simulink model "mainController19a"  (R2019a)
settings: Solver=ode3  StartTime=0  StopTime=inf  FixedStep=0.1  RelTol=1e-3
model workspace (MAT data in the model file):
  SL_ROS_VariableLengthArrays_MaxSizes : struct (value not decoded)
values from neighbouring files (symbols this model uses):
  numJoints = MotominiParams.numJoints    [showCompleteDemo.m]
  numPoints = size(Q,2)-2    [showCompleteDemo.m]
undefined symbols (not defined in the file or in its folder): homeToIdleSpline, idleToHomeSpline, Position, Position_SL_Info, Positions, Positions_SL_Info, TimeFromStart, Velocities, Velocities_SL_Info
libraries: robotlib x18, visiontextngfix x3, simulink x2, visionsinks x1
(part 2 of 2)

== matlab function mainController19a/Motion Planner/Planner Response/Joint Trajectory to Spline Matrices/pointsToSplineData ==
  data: pointsMsg input; Q output double size=[numJoints, numPoints+2]; dQ output double size=[numJoints, numPoints+2]; t output double size=[1, numPoints+2]; numJoints parameter; numPoints parameter; isValid output boolean size=[1]
function [Q,dQ,t, isValid] = pointsMsgToSplineData(pointsMsg,numJoints,numPoints)
% Author: Carlos Santacruz-Rosero, Ph.D.
% Copyright 2016 The MathWorks, Inc.

points = pointsMsg(1:numPoints+2);

Q = zeros(numJoints, numPoints+2);
dQ = zeros(numJoints, numPoints+2);
t = zeros(1,numPoints+2);
isValid = true;

numRxJoints = points(1).Positions_SL_Info.CurrentLength;

if numRxJoints ~= numJoints
    isValid = false;
end

for ii = 1:(numPoints+2)
    Q(:,ii) = points(ii).Positions(1:numJoints);
    dQ(:,ii) = points(ii).Velocities(1:numJoints);
    dur = points(ii).TimeFromStart;
    t(ii) =  double(dur.Sec)+double(dur.Nsec)*10^-9;
end

== stateflow chart mainController19a/State Controller/State Controller ==
  state Home
    state Home
      entry:
      requestTrajController = false;
      requestGripController = false;
      plannerRequest= false;
      droppingPos = [0.05;0.2;0.1];
      gripperOpenPos = [0.050; 0.050];
      gripperClosedPos =[0; 0];
    state GoingToHome
      entry:
      % move arm
      requestTrajController = true;
      Qspline = idleToHomeSpline.Q;
      dQspline = idleToHomeSpline.dQ;
      tSpline = idleToHomeSpline.t;
      goalSpline = idleToHomeSpline.Q(:,end);
      % close gripper
      requestGripController = true;
      gripCommand = [0; 0];
      during: % Going To Target
      requestTrajController = false;
      requestGripController = false;
    (default) -> Home.Home
    (junction 80) -> Home.Home
    GoingToHome -> (junction 80) : [goalReached && qActIsValid]
  state Idle
    state GoingToIdle
      entry:
      % move arm
      requestTrajController = true;
      Qspline = homeToIdleSpline.Q;
      dQspline = homeToIdleSpline.dQ;
      tSpline = homeToIdleSpline.t;
      goalSpline = homeToIdleSpline.Q(:,end);
      % open gripper
      requestGripController = true;
      gripCommand = gripperOpenPos;
      during: % Going To Target
      requestTrajController = false;
      requestGripController = false;
    state Idle
      entry:
      objectDetected = uint32(0);
      objectDetectedPos = zeros(3,1);
      % open gripper
      requestGripController = true;
      gripCommand = gripperOpenPos;
      during:
      [objectDetected, objectDetectedPos,droppingPos] = isObjectInScene(detectorPredictedLabels, detectorXYZPoints)
      requestGripController = false;
    GoingToIdle -> Idle.Idle : [goalReached && qActIsValid]
  state Grabbing
    state RequestGrabbingPlan
      entry:
      plannerRequest= true;
      requestTrajController=false;
      plannerObjectID = objectDetected;
      plannerPos = [objectDetectedPos(1);
      objectDetectedPos(2);
      0.018];
      during:
      plannerRequest= false;
      exit:
    state GoingToApproachPoint
      entry:
      requestTrajController = true;
      Qspline = plannerQ;
      dQspline = plannerDQ;
      tSpline = plannerT;
      goalSpline = plannerQ(:,end);
      during: % Going To Target
      requestTrajController = false;
    state RequestApproachingPlan
      entry:
      plannerRequest= true;
      plannerObjectID = objectDetected;
      plannerPos = [objectDetectedPos(1);
      objectDetectedPos(2);
      objectDetectedPos(3)+0.03];
      during:
      plannerRequest= false;
    state DroppingObject
      entry:
      requestGripController = true;
      gripCommand = gripperOpenPos;
      during: % Going To Target
      requestGripController = false;
    state GoingToObject
      entry:
      requestTrajController = true;
      Qspline = plannerQ;
      dQspline = plannerDQ;
      tSpline = plannerT;
      goalSpline = plannerQ(:,end);
      during: % Going To Target
      requestTrajController = false;
    state RequestLeavingPlan
      entry:
      plannerRequest= true;
      plannerObjectID = objectDetected;
      plannerPos = [objectDetectedPos(1);
      objectDetectedPos(2);
      objectDetectedPos(3)+0.1];
      during:
      plannerRequest= false;
      exit:
    state GrabbingObject
      entry:
      gripCommand = gripperClosedPos;
      requestGripController = true;
      during: % Going To Target
      requestGripController = false;
    state GoingToLeavingPoint
      entry:
      requestTrajController = true;
      Qspline = plannerQ;
      dQspline = plannerDQ;
      tSpline = plannerT;
      goalSpline = plannerQ(:,end);
      during: % Going To Leaving Point
      requestTrajController = false;
    state GoingToDroppingPoint
      entry:
      requestTrajController = true;
      Qspline = plannerQ;
      dQspline = plannerDQ;
      tSpline = plannerT;
      goalSpline = plannerQ(:,end);
      during: % Going To Target
      requestTrajController = false;
    state RequestDroppingPlan
      entry:
      plannerRequest= true;
      plannerObjectID = objectDetected;
      plannerPos = droppingPos;
      during:
      plannerRequest= false;
    RequestGrabbingPlan -> GoingToObject : [plannerHasReplied && ...
        | plannerIsValid]
    RequestApproachingPlan -> GoingToApproachPoint : [plannerHasReplied && ...
        | plannerIsValid]
    GoingToApproachPoint -> RequestGrabbingPlan : [goalReached && qActIsValid]
    GoingToDroppingPoint -> DroppingObject : [goalReached && qActIsValid]
    GoingToObject -> GrabbingObject : [goalReached && qActIsValid]
    GrabbingObject -> RequestLeavingPlan : [~isGripperOpen]
    RequestLeavingPlan -> GoingToLeavingPoint : [plannerHasReplied && ...
        | plannerIsValid]
    RequestDroppingPlan -> GoingToDroppingPoint : [plannerHasReplied && ...
        | plannerIsValid]
    GoingToLeavingPoint -> RequestDroppingPlan : [goalReached && qActIsValid]
  Home.Home -> Idle.Idle : [armCommand==1]
  (default) -> Home
  DroppingObject -> GoingToIdle : [isGripperOpen]
  Idle.Idle -> GoingToHome [order 1] : [armCommand == 0]
  Idle.Idle -> RequestApproachingPlan [order 2] : [(objectDetected ~=0) && qActIsValid]
  data: objDetected function_output uint32; objPos function_output; labels function_input uint32; points function_input double; dropPos function_output; armCommand input uint32; detectorPredictedLabels input uint32 size=[10 1]; detectorXYZPoints input double size=[10 3]; plannerHasReplied input boolean size=[1]; plannerQ input double; plannerDQ input double; plannerT input double; plannerIsValid input boolean; qActIsValid input boolean; plannerRequest output boolean size=[1]; plannerPos output double size=[3]; plannerObjectID output uint32 size=[1]; requestTrajController output boolean size=[1]; Qspline output double; dQspline output double; tSpline output; goalReached input boolean; homeToIdleSpline parameter; idleToHomeSpline parameter; requestGripController output boolean; gripCommand output double size=[2 1]; goalSpline output double size=[numJoints,1] =zeros(numJoints,1); gripperOpenPos local =[0.025;0.025]; gripperClosedPos local =[0;0]; droppingPos local; objectDetected local uint32 size=[1]; objectDetectedPos local double size=[3]; data1 local; isGripperOpen input
  function [objDetected,objPos,dropPos] = isObjectInScene(labels, points):
    | function [objDetected,objPos,dropPos] = isObjectInScene(labels, points)
    | 
    | objDetected = uint32(0);
    | objPos = zeros(3,1);
    | dropPositions = [0.00 0.2 0.1; 0.15 0.2 0.1; 0.30 0.2 0.1];
    | dropPos = zeros(3,1);
    |     
    | if ~isempty(labels)
    |     maxLabels = length(labels);
    |     %for ii =1:maxLabels
    |        %if objToGrab == labels(ii)
    |            objDetected = labels(1);
    |            objPos(1:3,1) = points(1,:)';
    |            % Compensate estimation error:
    | %           objPos(3,1) = objPos(3,1) - 0.05;
    |            objPos(1,1) = objPos(1,1) - 0.01;
    | %            objPos(2,1) = objPos(2,1) + 0.025;
    | %           objPos(3,1) = objPos(3,1);
    | %           objPos(1,1) = objPos(1,1);
    | %           objPos(2,1) = objPos(2,1);
    |            %return;
    |        %end
    |     %end
    |     dropPos = dropPositions(objDetected,:)';
    | end

== matlab function mainController19a/Object Detector/Display/Formatting ==
  data: predictedLabels input size=[10 1]; Variables output size=[5 10]; xyzPoints input size=[10 3]; Color output size=[10 3]; Location output size=[10 2]
function [Variables,Color,Location] = concatenateVectors(predictedLabels,xyzPoints)
%#codegen
    Variables = single([1:size(predictedLabels,1); predictedLabels'; xyzPoints']);
    Color = ones(size(predictedLabels,1),3,'single');
    Location = [zeros(size(predictedLabels,1),1,'single') single((0:(size(predictedLabels,1)-1))'*25)];

== matlab function mainController19a/Object Detector/Display/MATLAB Function ==
  data: u input size=[10 1]; y output size=[10 1]
function y = genSequence(u) %#codegen
    y = int32(find(u));

== matlab function mainController19a/Robot ROS Interface1/Arm Trajectory Controller/ Assign Joint Trajectory ==
  data: blankMessage input; jointTrajPoints input; msg output Bus: SL_Bus_mainController_trajectory_msgs_JointTrajectory
function msg = assignJointTrajectory(blankMessage, jointTrajPoints)
%#codegen

% To set datatype of MSG output:
%  1. Create buses for this model: robotics.ros.createSimulinkBus(gcs)
%  1. Click "Edit Data" in  Toolstrip to open "Ports and Data Manager"
%  2. Select MSG and set datatype to "Bus: SL_Bus_<modelname>_<messageType>"
% See:
% http://www.mathworks.com/help/simulink/ug/create-structures-in-matlab-function-blocks.html


% Assign string array with joint names:
strArrayToAssign = {'joint_1_s',...
    'joint_2_l',...
    'joint_3_u',...
    'joint_4_r',...
    'joint_5_b',...
    'joint_6_t'};

% Assign Joint Trajectory Point:
numPoints = size(jointTrajPoints,1);
blankMessage.Points_SL_Info.CurrentLength = uint32(numPoints);
for ii = 1:numPoints
    blankMessage.Points(ii) = jointTrajPoints(ii);
end

numStringsInArray = length(strArrayToAssign);
blankMessage.JointNames_SL_Info.CurrentLength = uint32(numStringsInArray);

for idx=1:numStringsInArray
    str = strArrayToAssign{idx};
    strLength = length(str);
    blankMessage.JointNames(idx).Data(1:strLength) = uint8(str);
    blankMessage.JointNames(idx).Data_SL_Info.CurrentLength = uint32(strLength);
end

msg = blankMessage;

== matlab function mainController19a/Robot ROS Interface1/Gripper Trajectory Controller/ Assign Joint Trajectory ==
  data: blankMessage input; jointTrajPoints input; msg output Bus: SL_Bus_mainController_trajectory_msgs_JointTrajectory
function msg = assignJointTrajectory(blankMessage, jointTrajPoints)
%#codegen

% To set datatype of MSG output:
%  1. Create buses for this model: robotics.ros.createSimulinkBus(gcs)
%  1. Click "Edit Data" in  Toolstrip to open "Ports and Data Manager"
%  2. Select MSG and set datatype to "Bus: SL_Bus_<modelname>_<messageType>"
% See: 
% http://www.mathworks.com/help/simulink/ug/create-structures-in-matlab-function-blocks.html


% Assign string array with joint names:
strArrayToAssign = {'gripper_finger_joint_l'; 'gripper_finger_joint_r'};

% Assign Joint Trajectory Point:
numPoints = size(jointTrajPoints,1);
blankMessage.Points_SL_Info.CurrentLength = uint32(numPoints);
for ii = 1:numPoints
    blankMessage.Points(ii) = jointTrajPoints(ii);
end

numStringsInArray = length(strArrayToAssign);
blankMessage.JointNames_SL_Info.CurrentLength = uint32(numStringsInArray);

for idx=1:numStringsInArray
    str = strArrayToAssign{idx};
    strLength = length(str);
    blankMessage.JointNames(idx).Data(1:strLength) = uint8(str);
    blankMessage.JointNames(idx).Data_SL_Info.CurrentLength = uint32(strLength);
end

msg = blankMessage;
